simulink model "textf23"  (R2021b)
settings: Solver=FixedStepAuto  StartTime=0.0  StopTime=10  FixedStep=0.01  RelTol=1e-3
libraries: simulink x5
settings Model: Creator=asus  LastModifiedBy=asus

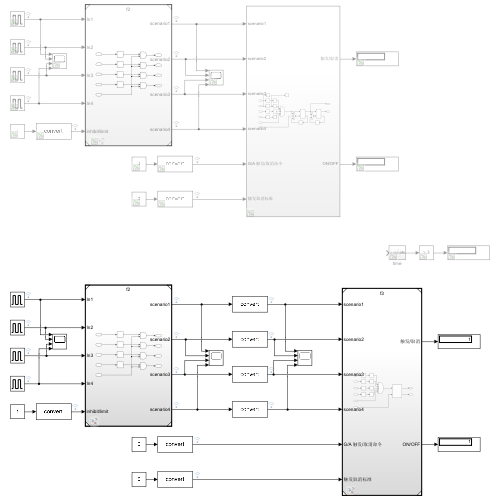
[thumbnail: Simulink's stored preview of the top-level diagram]
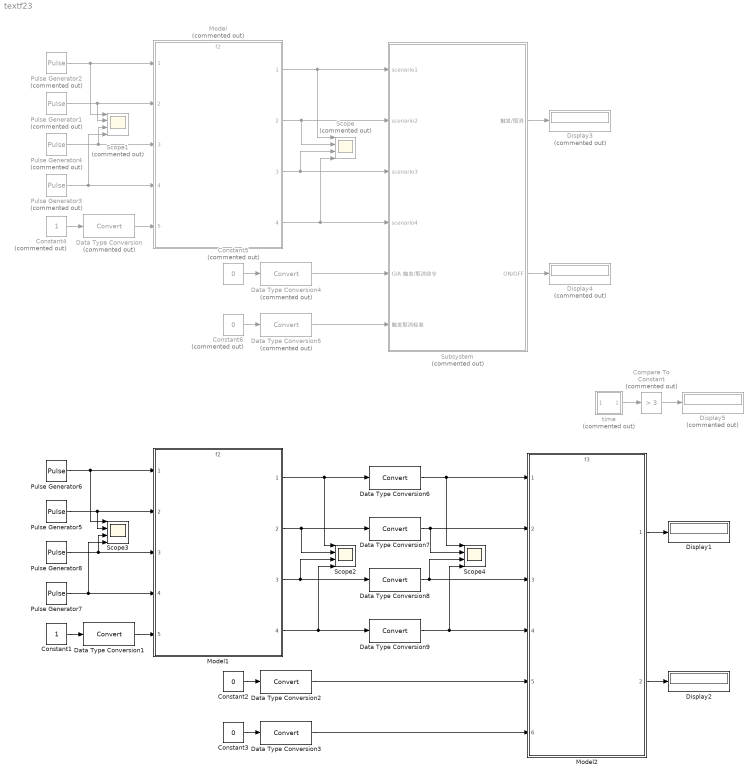
== system textf23 ==
  Compare To Constant : simulink/Logic and Bit Operations/Compare To Constant  Commented=on  relop=>  const=3  OutDataTypeStr=boolean
  Constant1 : Constant
  Constant2 : Constant  Value=0
  Constant3 : Constant  Value=0
  Constant4 : Constant  Commented=on
  Constant5 : Constant  Commented=on  Value=0
  Constant6 : Constant  Commented=on  Value=0
  Data Type Conversion : DataTypeConversion  Commented=on
  Data Type Conversion{1..3,6..9} (7 alike) : DataTypeConversion
  Data Type Conversion4 : DataTypeConversion  Commented=on
  Data Type Conversion5 : DataTypeConversion  Commented=on
  Display1 : Display
  Display2 : Display
  Display3 : Display  Commented=on
  Display4 : Display  Commented=on
  Display5 : Display  Commented=on
  Model : ModelReference  Commented=on  ModelNameDialog=f2.slx  SimulationMode=Normal  ModelReferenceVersion=1.6
  Model1 : ModelReference  ModelNameDialog=f2.slx  SimulationMode=Normal  ModelReferenceVersion=1.7
  Model2 : ModelReference  ModelNameDialog=f3.slx  SimulationMode=Normal  ModelReferenceVersion=1.17
  Pulse Generator1 : DiscretePulseGenerator  Commented=on  PulseType=Time based  Amplitude=5  Period=10  PulseWidth=50
  Pulse Generator2 : DiscretePulseGenerator  Commented=on  PulseType=Time based  Amplitude=2  Period=10  PulseWidth=50
  Pulse Generator3 : DiscretePulseGenerator  Commented=on  PulseType=Time based  Amplitude=0  Period=10  PulseWidth=50
  Pulse Generator4 : DiscretePulseGenerator  Commented=on  PulseType=Time based  Amplitude=5  Period=10  PulseWidth=20
  Pulse Generator5 : DiscretePulseGenerator  PulseType=Time based  Amplitude=5  Period=10  PulseWidth=50
  Pulse Generator6 : DiscretePulseGenerator  PulseType=Time based  Amplitude=2  Period=10  PulseWidth=50
  Pulse Generator7 : DiscretePulseGenerator  PulseType=Time based  Amplitude=0  Period=10  PulseWidth=50
  Pulse Generator8 : DiscretePulseGenerator  PulseType=Time based  Amplitude=5  Period=10  PulseWidth=20
  Scope : Scope  Commented=on  NumInputPorts=4
  Scope1 : Scope  Commented=on  NumInputPorts=4
  Scope2 : Scope  NumInputPorts=4
  Scope3 : Scope  NumInputPorts=4
  Scope4 : Scope  NumInputPorts=4
  Subsystem : Subsystem  Commented=on
  time : Subsystem  Commented=on
  wires:
  Pulse Generator2/1 -> Scope1/1, Model/1
  Pulse Generator1/1 -> Scope1/2, Model/2
  Pulse Generator4/1 -> Scope1/3, Model/3
  Pulse Generator3/1 -> Scope1/4, Model/4
  Constant4/1 -> Data Type Conversion/1
  Data Type Conversion/1 -> Model/5
  Model/1 -> Scope/1, Subsystem/1(scenario1)
  Model/3 -> Scope/3, Subsystem/3(scenario3)
  Model/4 -> Scope/4, Subsystem/4(scenario4)
  Model/2 -> Scope/2, Subsystem/2(scenario2)
  Constant5/1 -> Data Type Conversion4/1
  Constant6/1 -> Data Type Conversion5/1
  Data Type Conversion4/1 -> Subsystem/5(G/A 触发/取消命令)
  Data Type Conversion5/1 -> Subsystem/6(触发取消标准)
  Subsystem/1(触发/取消) -> Display3/1
  Subsystem/2(ON/OFF) -> Display4/1
  Pulse Generator8/1 -> Scope3/3, Model1/3
  Pulse Generator6/1 -> Scope3/1, Model1/1
  Pulse Generator5/1 -> Scope3/2, Model1/2
  Model1/3 -> Data Type Conversion8/1, Scope2/3
  Model1/1 -> Scope2/1, Data Type Conversion6/1
  Constant1/1 -> Data Type Conversion1/1
  Data Type Conversion1/1 -> Model1/5
  Constant2/1 -> Data Type Conversion2/1
  Pulse Generator7/1 -> Scope3/4, Model1/4
  Model1/4 -> Scope2/4, Data Type Conversion9/1
  Model2/2 -> Display2/1
  Model1/2 -> Scope2/2, Data Type Conversion7/1
  Model2/1 -> Display1/1
  Data Type Conversion2/1 -> Model2/5
  Constant3/1 -> Data Type Conversion3/1
  Data Type Conversion3/1 -> Model2/6
  Data Type Conversion7/1 -> Model2/2, Scope4/2
  Data Type Conversion9/1 -> Scope4/4, Model2/4
  Data Type Conversion6/1 -> Model2/1, Scope4/1
  Data Type Conversion8/1 -> Model2/3, Scope4/3
  time/1(Out1) -> Compare To Constant/1
  Compare To Constant/1 -> Display5/1

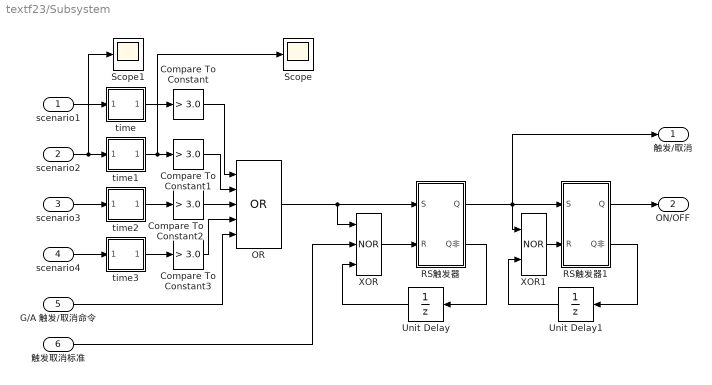
== system textf23/Subsystem ==
  scenario1 : Inport
  scenario2 : Inport  Port=2
  scenario3 : Inport  Port=3
  scenario4 : Inport  Port=4
  G/A 触发/取消命令 : Inport  Port=5
  触发取消标准 : Inport  Port=6
  Compare To Constant{,1..3} (4 alike) : simulink/Logic and Bit Operations/Compare To Constant  relop=>  const=3.0  OutDataTypeStr=boolean
  OR : Logic  Operator=OR  Inputs=5  IconShape=distinctive  AllPortsSameDT=off  OutDataTypeStr=boolean
  RS触发器 : Subsystem
  RS触发器1 : Subsystem
  Scope : Scope
  Scope1 : Scope
  Unit Delay : UnitDelay  SampleTime=-1  HasFrameUpgradeWarning=on
  Unit Delay1 : UnitDelay  SampleTime=-1  HasFrameUpgradeWarning=on
  XOR : Logic  Operator=NOR  Inputs=3  IconShape=distinctive  AllPortsSameDT=off  OutDataTypeStr=boolean
  XOR1 : Logic  Operator=NOR  IconShape=distinctive  AllPortsSameDT=off  OutDataTypeStr=boolean
  time : Subsystem
  time1 : Subsystem
  time2 : Subsystem
  time3 : Subsystem
  触发/取消 : Outport
  ON/OFF : Outport  Port=2
  wires:
  time2/1(Out1) -> Compare To Constant2/1
  OR/1 -> RS触发器/1(S), XOR/1
  scenario3/1 -> time2/1(scenario3)
  time3/1(Out1) -> Compare To Constant3/1
  time1/1(Out1) -> Scope/1, Compare To Constant1/1
  G/A 触发/取消命令/1 -> OR/5
  Compare To Constant1/1 -> OR/2
  XOR1/1 -> RS触发器1/2(R)
  Compare To Constant3/1 -> OR/4
  Compare To Constant2/1 -> OR/3
  Unit Delay/1 -> XOR/3
  RS触发器1/2(Q非) -> Unit Delay1/1
  Compare To Constant/1 -> OR/1
  time/1(Out1) -> Compare To Constant/1
  XOR/1 -> RS触发器/2(R)
  Unit Delay1/1 -> XOR1/2
  触发取消标准/1 -> XOR/2
  scenario1/1 -> time/1(scenario1)
  scenario4/1 -> time3/1(scenario4)
  scenario2/1 -> Scope1/1, time1/1(scenario2)
  RS触发器1/1(Q) -> ON/OFF/1
  RS触发器/1(Q) -> XOR1/1, 触发/取消/1, RS触发器1/1(S)
  RS触发器/2(Q非) -> Unit Delay/1

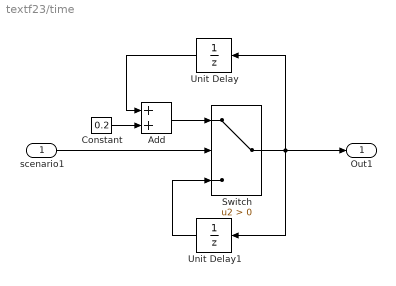
== system textf23/time ==
  scenario1 : Inport
  Add : Sum
  Constant : Constant  Value=0.2
  Switch : Switch  Criteria=u2 > Threshold
  Unit Delay : UnitDelay  SampleTime=-1  HasFrameUpgradeWarning=on
  Unit Delay1 : UnitDelay  SampleTime=-1  HasFrameUpgradeWarning=on
  Out1 : Outport
  wires:
  scenario1/1 -> Switch/2
  Unit Delay/1 -> Add/1
  Switch/1 -> Out1/1, Unit Delay/1, Unit Delay1/1
  Constant/1 -> Add/2
  Add/1 -> Switch/1
  Unit Delay1/1 -> Switch/3

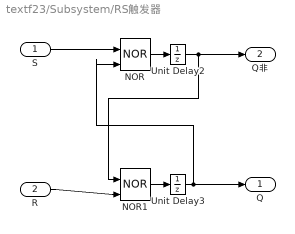
== system textf23/Subsystem/RS触发器 ==
  S : Inport
  R : Inport  Port=2
  NOR : Logic  Operator=NOR  IconShape=distinctive  AllPortsSameDT=off  OutDataTypeStr=boolean
  NOR1 : Logic  Operator=NOR  IconShape=distinctive  AllPortsSameDT=off  OutDataTypeStr=boolean
  Unit Delay2 : UnitDelay  SampleTime=-1  HasFrameUpgradeWarning=on
  Unit Delay3 : UnitDelay  SampleTime=-1  HasFrameUpgradeWarning=on
  Q : Outport
  Q非 : Outport  Port=2
  wires:
  S/1 -> NOR/1
  R/1 -> NOR1/2
  NOR1/1 -> Unit Delay3/1
  NOR/1 -> Unit Delay2/1
  Unit Delay2/1 -> NOR1/1, Q非/1
  Unit Delay3/1 -> NOR/2, Q/1

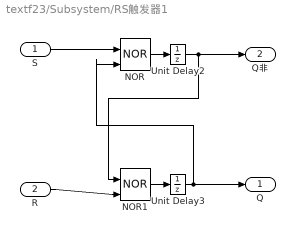
== system textf23/Subsystem/RS触发器1 ==
  S : Inport
  R : Inport  Port=2
  NOR : Logic  Operator=NOR  IconShape=distinctive  AllPortsSameDT=off  OutDataTypeStr=boolean
  NOR1 : Logic  Operator=NOR  IconShape=distinctive  AllPortsSameDT=off  OutDataTypeStr=boolean
  Unit Delay2 : UnitDelay  SampleTime=-1  HasFrameUpgradeWarning=on
  Unit Delay3 : UnitDelay  SampleTime=-1  HasFrameUpgradeWarning=on
  Q : Outport
  Q非 : Outport  Port=2
  wires:
  Unit Delay3/1 -> Q/1, NOR/2
  Unit Delay2/1 -> Q非/1, NOR1/1
  NOR/1 -> Unit Delay2/1
  NOR1/1 -> Unit Delay3/1
  R/1 -> NOR1/2
  S/1 -> NOR/1

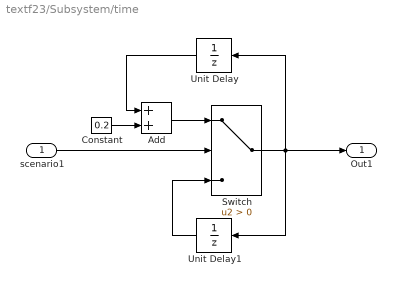
== system textf23/Subsystem/time ==
  scenario1 : Inport
  Add : Sum
  Constant : Constant  Value=0.2
  Switch : Switch  Criteria=u2 > Threshold
  Unit Delay : UnitDelay  SampleTime=-1  HasFrameUpgradeWarning=on
  Unit Delay1 : UnitDelay  SampleTime=-1  HasFrameUpgradeWarning=on
  Out1 : Outport
  wires:
  scenario1/1 -> Switch/2
  Unit Delay/1 -> Add/1
  Switch/1 -> Out1/1, Unit Delay/1, Unit Delay1/1
  Constant/1 -> Add/2
  Add/1 -> Switch/1
  Unit Delay1/1 -> Switch/3

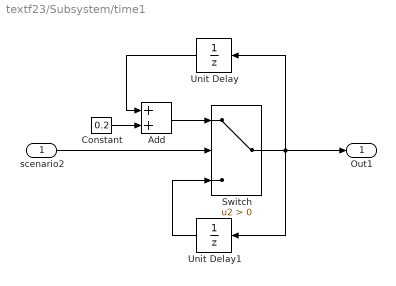
== system textf23/Subsystem/time1 ==
  scenario2 : Inport
  Add : Sum
  Constant : Constant  Value=0.2
  Switch : Switch  Criteria=u2 > Threshold
  Unit Delay : UnitDelay  SampleTime=-1  HasFrameUpgradeWarning=on
  Unit Delay1 : UnitDelay  SampleTime=-1  HasFrameUpgradeWarning=on
  Out1 : Outport
  wires:
  Unit Delay1/1 -> Switch/3
  Add/1 -> Switch/1
  Constant/1 -> Add/2
  Switch/1 -> Unit Delay1/1, Unit Delay/1, Out1/1
  Unit Delay/1 -> Add/1
  scenario2/1 -> Switch/2

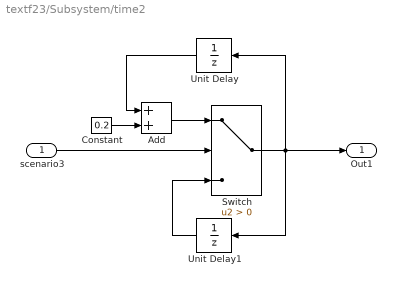
== system textf23/Subsystem/time2 ==
  scenario3 : Inport
  Add : Sum
  Constant : Constant  Value=0.2
  Switch : Switch  Criteria=u2 > Threshold
  Unit Delay : UnitDelay  SampleTime=-1  HasFrameUpgradeWarning=on
  Unit Delay1 : UnitDelay  SampleTime=-1  HasFrameUpgradeWarning=on
  Out1 : Outport
  wires:
  Unit Delay1/1 -> Switch/3
  Add/1 -> Switch/1
  Constant/1 -> Add/2
  Switch/1 -> Unit Delay1/1, Unit Delay/1, Out1/1
  Unit Delay/1 -> Add/1
  scenario3/1 -> Switch/2

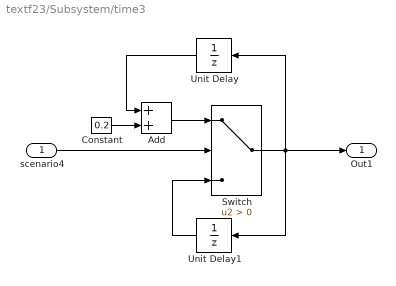
== system textf23/Subsystem/time3 ==
  scenario4 : Inport
  Add : Sum
  Constant : Constant  Value=0.2
  Switch : Switch  Criteria=u2 > Threshold
  Unit Delay : UnitDelay  SampleTime=-1  HasFrameUpgradeWarning=on
  Unit Delay1 : UnitDelay  SampleTime=-1  HasFrameUpgradeWarning=on
  Out1 : Outport
  wires:
  scenario4/1 -> Switch/2
  Unit Delay/1 -> Add/1
  Switch/1 -> Out1/1, Unit Delay/1, Unit Delay1/1
  Constant/1 -> Add/2
  Add/1 -> Switch/1
  Unit Delay1/1 -> Switch/3
